simulink model "sim_ekf_est_motor_3para"  (R2020b)
settings: Solver=ode1  StartTime=0.0  StopTime=100  FixedStep=0.01  RelTol=1e-3
undefined symbols (not defined in the file): DiscIntNeverNeededParam
settings Model: Creator=Admin  LastModifiedBy=ONLY-GOD

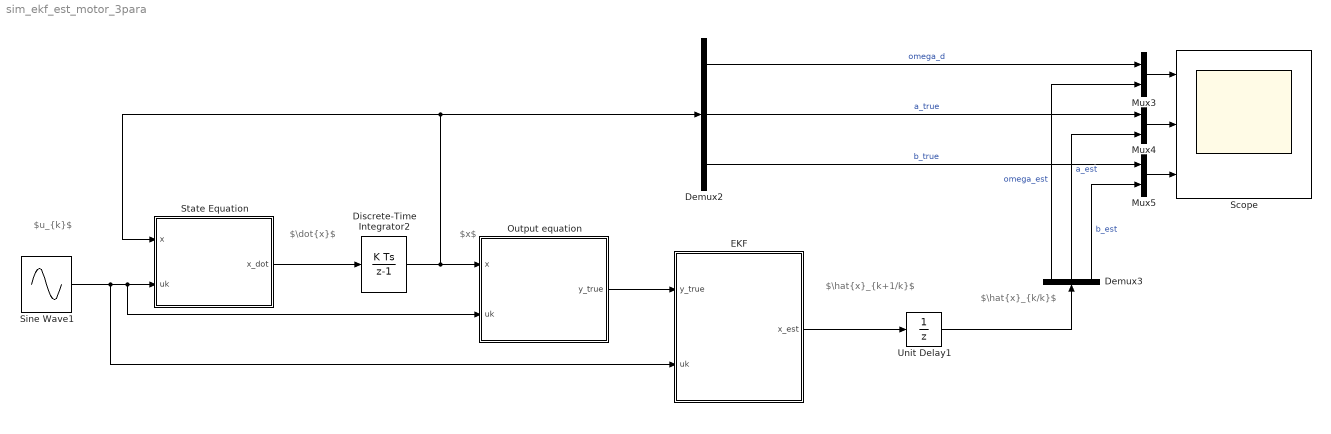
== system sim_ekf_est_motor_3para ==
  note: $x$
  note: $\hat{x}_{k+1/k}$
  note: $\hat{x}_{k/k}$
  note: $\dot{x}$
  note: $u_{k}$
  Demux2 : Demux  Outputs=3
  Demux3 : Demux  Outputs=3
  Discrete-Time Integrator2 : DiscreteIntegrator  InitialCondition=[0;20;40]  SampleTime=-1  ICPrevOutput=DiscIntNeverNeededParam  ICPrevScaledInput=DiscIntNeverNeededParam
  EKF : MATLAB Function  TreatAsAtomicUnit=on
  Mux3 : Mux  Inputs=2
  Mux4 : Mux  Inputs=2
  Mux5 : Mux  Inputs=2
  Output equation : MATLAB Function  TreatAsAtomicUnit=on
  Scope : Scope  NumInputPorts=3
  Sine Wave1 : Sin  Amplitude=20  Frequency=2*pi*0.1  SampleTime=0
  State Equation : MATLAB Function  TreatAsAtomicUnit=on
  Unit Delay1 : UnitDelay  InitialCondition=[0;0;0]  SampleTime=-1  HasFrameUpgradeWarning=on
  wires:
  Mux4/1 -> Scope/2
  Mux5/1 -> Scope/3
  Mux3/1 -> Scope/1
  Demux2/1 -> Mux3/1  "omega_d"
  Demux2/2 -> Mux4/1  "a_true"
  Demux3/1 -> Mux3/2  "omega_est"
  Discrete-Time Integrator2/1 -> Output equation/1(x), State Equation/1(x), Demux2/1
  Demux3/3 -> Mux5/2  "b_est"
  EKF/1(x_est) -> Unit Delay1/1
  Demux2/3 -> Mux5/1  "b_true"
  Demux3/2 -> Mux4/2  "a_est"
  Unit Delay1/1 -> Demux3/1
  State Equation/1(x_dot) -> Discrete-Time Integrator2/1
  Sine Wave1/1 -> EKF/2(uk), Output equation/2(uk), State Equation/2(uk)
  Output equation/1(y_true) -> EKF/1(y_true)

== matlab function sim_ekf_est_motor_3para/Output equation ==
  settings: updateMethod=DISCRETE
  data: x input; uk input; y_true output
function y_true = output_eq(x,uk)
C = [1 0 0];
D = 0;
y_true = C*x+D*uk+sqrt(0.02)*randn;

== matlab function sim_ekf_est_motor_3para/EKF ==
  settings: updateMethod=DISCRETE
  data: y_true input; uk input; x_est output
function x_est = ekf(y_true, uk)
Ts = 0.01; %Time step
persistent x_est_p P Qd_est R_est Qc_est; % initialize initial value
if isempty(x_est_p)
    x_est_p = [0;0;0]; % initial value of x_est ( free to choose randomly )
    P       = 1e-4*diag([10,1,30]); % variance matrix
    Qc_est  = 1e-4*diag([1,10,100]); % process noise ( small = believe process )
    Qd_est  = Ts*Qc_est; % process noise decretized from process noise continuous
    R_est   = 0.001; % measurement noise ( small = believe measurement )
end
c  = [1 0 0];
D  = 0;
Ck = c;
Dk = D;

%Comput Kalman Gain and update predicted value
Wk    = P*Ck'/(Ck*P*Ck'+R_est);
y_est = Ck*x_est_p+Dk*uk;
x     = x_est_p+Wk.*(y_true-y_est);

%Compute prediction at next time step
x_est = x+Ts*[-x(2)*x(1)+uk*x(3);
                      0;
                      0];

%Update error covariance matrices
P = P-Wk*Ck*P;

%Define Ak
Ak      = eye(3)+Ts*[-x(2) -x(1) uk;
                       0     0    0;
                       0     0    0]; % jacobian matrix (deriative)
P       = Ak*P*Ak'+Qd_est;
x_est_p = x_est;

== matlab function sim_ekf_est_motor_3para/State Equation ==
  settings: updateMethod=DISCRETE
  data: x input; uk input; x_dot output
function x_dot = state_eq(x,uk)
x_dot = [0;0;0];
x_dot(1) = -x(1)*x(2)+x(3)*uk+sqrt(0.02)*sqrt(0.01)*randn;
x_dot(2) = 0;
x_dot(3) = 0;
